simulink model "breakfor"  (Simulink 6.4)
settings: Solver=FixedStepDiscrete  StartTime=0.0  StopTime=10.0  RelTol=1e-3
libraries: simulink x1
settings Model: Creator=bpatel  LastModifiedBy=bpatel

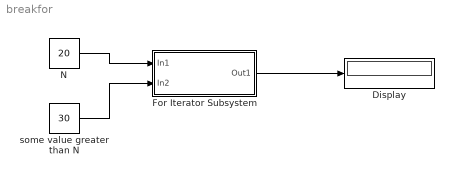
== system breakfor ==
  Display : Display
  For Iterator Subsystem : Subsystem  TreatAsAtomicUnit=on
  N : Constant  Value=20  OutDataType=sfix(16)  ConRadixGroup=Use specified scaling  OutScaling=2^0  SampleTime=inf  FramePeriod=inf
  some value greater than N : Constant  Value=30  OutDataType=sfix(16)  ConRadixGroup=Use specified scaling  OutScaling=2^0  SampleTime=inf  FramePeriod=inf
  wires:
  For Iterator Subsystem/1(Out1) -> Display/1
  N/1 -> For Iterator Subsystem/1(In1)
  some value greater than N/1 -> For Iterator Subsystem/2(In2)

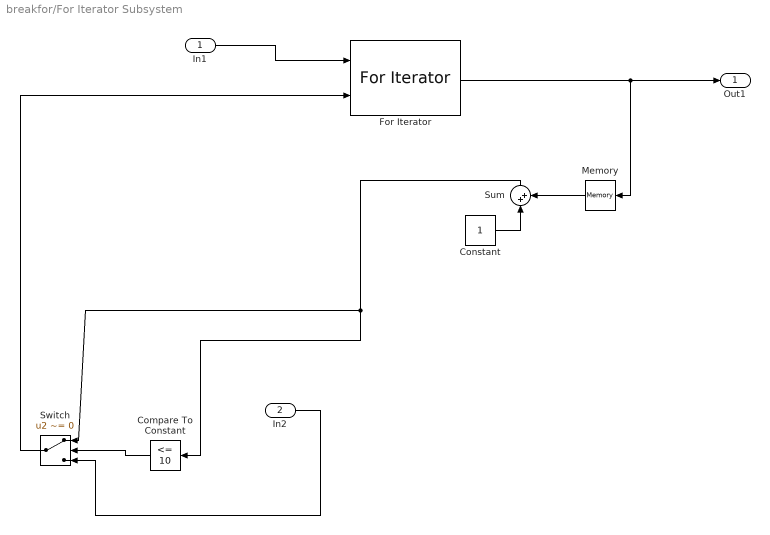
== system breakfor/For Iterator Subsystem ==
  In1 : Inport
  In2 : Inport  Port=2
  Compare To Constant : simulink/Logic and Bit Operations/Compare To Constant  Orientation=left  SystemSampleTime=-1  relop=<=  const=10  LogicOutDataTypeMode=uint8  ZeroCross=off
  Constant : Constant  Value=1  OutDataType=sfix(16)  ConRadixGroup=Use specified scaling  OutScaling=2^0  SampleTime=inf  FramePeriod=inf
  For Iterator : ForIterator  IterationSource=external  IterationLimit=20  ExternalIncrement=on  IterationVariableDataType=double
  Memory : Memory  Orientation=left  InheritSampleTime=on
  Sum : Sum  Orientation=up  Inputs=|++
  Switch : Switch  Orientation=left  Criteria=u2 ~= 0
  Out1 : Outport
  wires:
  Constant/1 -> Sum/1
  Memory/1 -> Sum/2
  For Iterator/1 -> Memory/1, Out1/1
  In2/1 -> Switch/3
  Compare To Constant/1 -> Switch/2
  Sum/1 -> Compare To Constant/1, Switch/1
  Switch/1 -> For Iterator/2
  In1/1 -> For Iterator/1
